simulink model "VTOL_renewal"  (R2023b)
settings: configuration reference "VTOLConfiguration" (kept outside this file)
undefined symbols (not defined in the file): CityMission, control, controlParams, ControlSampleTime, CriticalTiltAngle, DiscIntNeverNeededParam, env, F, FixedWingMission, flightState, FSState, FWControlParams, FWTrimSpeed, HoverMission, iniRoll, initPitch, iniYaw, Light, MIL, R_LOOKAHEAD, ReferenceFilterDen, ReferenceFilterNum, tilt_max, tilt_trim, tiltIni, TiltScheduleRate, TransitionMission, uavParam, vIni, Vt, w_trim, WindDownRate, windVel, xGround, yGround, zGround
libraries: slpidlib x56, simulink x6, uavalgslib x6, mbdriLib x4, aerolibasang x2, aerolibwind2 x2, shared6dof x1, sharedtransform x1, simulink_extras x1, sim3dlib x1, uavsim3dlib x1, uavutilslib x1
(part 1 of 8)
settings Model: DataDictionary=VTOLDynamicsData.sldd  Creator=The MathWorks, Inc.  LastModifiedBy=USER
settings ConfigSetRef: SourceName=VTOLConfiguration

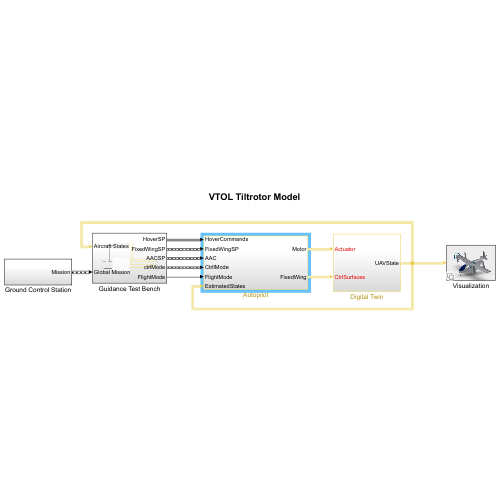
[thumbnail: Simulink's stored preview of the top-level diagram]
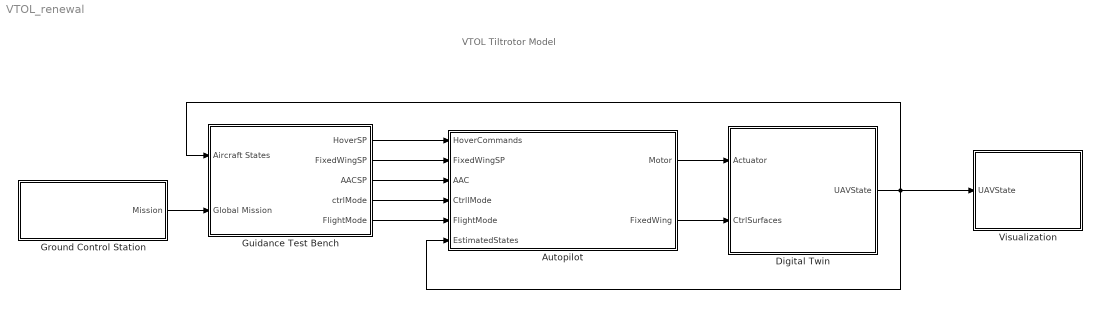
== system VTOL_renewal ==
  note: VTOL Tiltrotor Model
  Autopilot : Subsystem
  Digital Twin : Subsystem
  Ground Control Station : Subsystem
  Guidance Test Bench : Subsystem
  Visualization : Subsystem  Variant=on  VariantControl=Visualization
      mask Display: image('TiltrotorVisualization.PNG'); % Use "Edit Image" on toolstrip to change.
  wires:
  Autopilot/1(Motor) -> Digital Twin/1(Actuator)
  Autopilot/2(FixedWing) -> Digital Twin/2(CtrlSurfaces)
  Guidance Test Bench/1(HoverSP) -> Autopilot/1(HoverCommands)
  Ground Control Station/1(Mission) -> Guidance Test Bench/2(Global Mission)
  Guidance Test Bench/2(FixedWingSP) -> Autopilot/2(FixedWingSP)
  Guidance Test Bench/3(AACSP) -> Autopilot/3(AAC)
  Guidance Test Bench/5(FlightMode) -> Autopilot/5(FlightMode)
  Digital Twin/1(UAVState) -> Guidance Test Bench/1(Aircraft States), Autopilot/6(EstimatedStates), Visualization/1(UAVState)
  Guidance Test Bench/4(ctrlMode) -> Autopilot/4(CtrllMode)

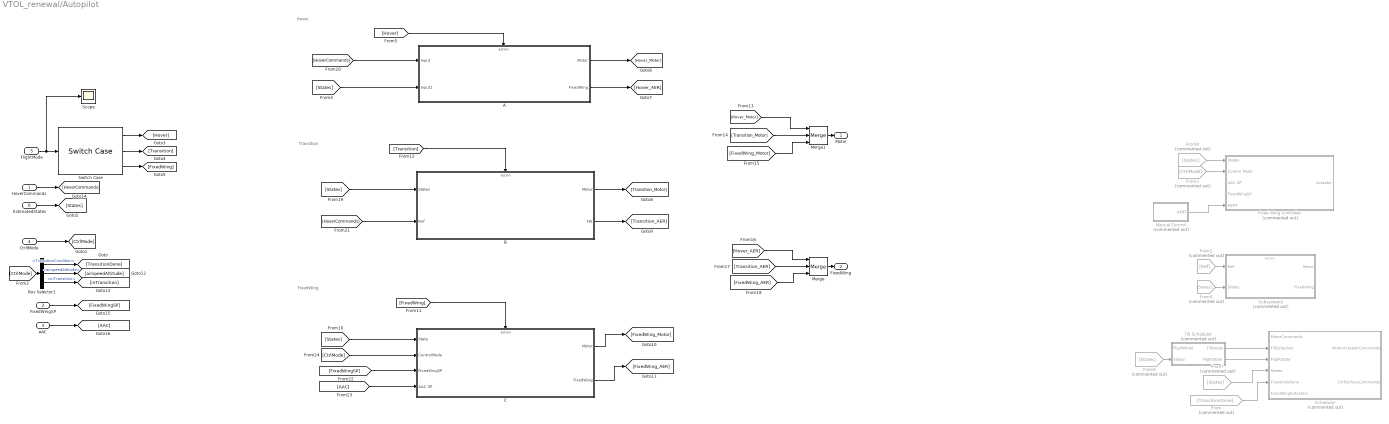
== system VTOL_renewal/Autopilot ==
  note: FixedWing
  note: Transition
  note: Hover
  HoverCommands : Inport
  FixedWingSP : Inport  Port=2
  AAC : Inport  Port=3
  CtrllMode : Inport  Port=4
  FlightMode : Inport  Port=5
  EstimatedStates : Inport  Port=6
  A : Subsystem  TreatAsAtomicUnit=on
  B : Subsystem
  Bus Selector1 : BusSelector  OutputSignals=TransitionCondition,airspeedAltitude,inTransition
  C : Subsystem
  Fixed Wing Controller : Subsystem  Commented=on  Variant=on  VariantControl=Fixed Wing Controller
  From : From  Commented=on  GotoTag=TransitionDone
  From1 : From  Commented=on  GotoTag=Ref
  From3 : From  Commented=on  GotoTag=CtrlMode
  From{6..9} (4 alike) : From  Commented=on  GotoTag=States
  Manual Control : Subsystem  Commented=on
  Merge : Merge  Inputs=3
  Merge1 : Merge  Inputs=3
  Scheduler : Subsystem  Commented=on  SystemSampleTime=0.005
  Scope : Scope
  Subsystem5 : Subsystem  Commented=on
  Switch Case : SwitchCase  CaseConditions={flightState.Hover, flightState.Transition, flightState.FixedWing}  ShowDefaultCase=off
  Tilt Scheduler : Subsystem  Commented=on
  Motor : Outport  OutDataTypeStr=Bus: RotorCntrlBus
  FixedWing : Outport  Port=2
  wires:
  Tilt Scheduler/1(TiltAngle) -> Scheduler/2(TiltSchedule)
  Manual Control/1(AERT) -> Fixed Wing Controller/5(AERT)
  From/1 -> Scheduler/5(TransitionDone)
  Tilt Scheduler/2(FlightState) -> Scheduler/3(FlightState)
  Bus Selector1/1 -> [TransitionDone]  "<TransitionCondition>"
  From3/1 -> Fixed Wing Controller/2(Control Mode)
  [CtrlMode] -> Bus Selector1/1
  EstimatedStates/1 -> [States]
  From8/1 -> Fixed Wing Controller/1(States)
  From6/1 -> Tilt Scheduler/2(States)
  From7/1 -> Scheduler/4(States)
  FlightMode/1 -> Scope/1, Switch Case/1
  Switch Case/1 -> [Hover]
  Switch Case/2 -> [Transition]
  Switch Case/3 -> [FixedWing]
  CtrllMode/1 -> [CtrlMode]
  From9/1 -> Subsystem5/2(States)
  From1/1 -> Subsystem5/1(Ref)
  [States] -> C/1(State)
  [Hover] -> A/Action
  [States] -> A/2(Input1)
  [Transition] -> B/Action
  A/1(Motor) -> [Hover_Motor]
  A/2(FixedWing) -> [Hover_AER]
  B/1(Motor) -> [Transition_Motor]
  B/2(FW) -> [Transition_AER]
  C/1(Motor) -> [FixedWing_Motor]
  C/2(FixedWing) -> [FixedWing_AER]
  [Transition_Motor] -> Merge1/2
  [Transition_AER] -> Merge/2
  [States] -> B/1(States)
  [FixedWing] -> C/Action
  Bus Selector1/2 -> [airspeedAltitude]  "<airspeedAltitude>"
  Bus Selector1/3 -> [inTransition]  "<inTransition>"
  FixedWingSP/1 -> [FixedWingSP]
  [Hover_Motor] -> Merge1/1
  [Hover_AER] -> Merge/1
  HoverCommands/1 -> [HoverCommands]
  [HoverCommands] -> A/1(Input)
  [HoverCommands] -> B/2(Ref)
  AAC/1 -> [AAC]
  [AAC] -> C/4(AAC SP)
  [FixedWingSP] -> C/3(FixedWingSP)
  [CtrlMode] -> C/2(ControlMode)
  Merge1/1 -> Motor/1
  [FixedWing_Motor] -> Merge1/3
  Merge/1 -> FixedWing/1
  [FixedWing_AER] -> Merge/3

== system VTOL_renewal/Digital Twin ==
  Actuator : Inport
  CtrlSurfaces : Inport  Port=2
  6DOF (Euler Angles)1 : shared6dof/6DOF (Euler Angles)  units=Metric (MKS)  mtype=Fixed  rep=Euler Angles  xme_0=[xGround, yGround, zGround]  Vm_0=[vIni 0 0]  eul_0=[iniRoll initPitch iniYaw]  pm_0=[0 0 0]  mass_0=6.031  mass_e=0.5  mass_f=2.0  inertia=[uavParam.geom.Ixx 0 0; 0 uavParam.geom.Iyy 0; 0 0 uavParam.geom.Izz]  inertia_e=eye(3)  inertia_f=2*eye(3)  k_quat=1.0  vre_flag=on  abi_flag=on  aMode=0  xme_statename=''  Vm_statename=''  eul_statename=''  quat_statename=''  pm_statename=''  mass_statename=''
  Bus Selector : BusSelector  OutputSignals=RotorParameters.w1,RotorParameters.w2,RotorParameters.w3,RotorParameters.w4
  Bus Selector1 : BusSelector  OutputSignals=Xe,Ve,Euler,pqr
  Demux : Demux  Outputs=3
  Demux1 : Demux  Outputs=3
  Force and Moments : Subsystem
  Ground Truth Bus : Subsystem
  Scope : Scope  NumInputPorts=4
  Scope{1..10} (10 alike) : Scope
  Subsystem2 : Subsystem
  Terminator : Terminator
  UAVState : Outport
  wires:
  Force and Moments/1(F) -> 6DOF (Euler Angles)1/1
  Force and Moments/2(M) -> 6DOF (Euler Angles)1/2
  Actuator/1 -> Force and Moments/1(Actuator)
  CtrlSurfaces/1 -> Force and Moments/2(CtrlSurfaces)
  6DOF (Euler Angles)1/1 -> Ground Truth Bus/1(Ve)  "Ve"
  6DOF (Euler Angles)1/2 -> Ground Truth Bus/2(Xe)  "Xe"
  6DOF (Euler Angles)1/3 -> Ground Truth Bus/3(Euler)  "Euler"
  6DOF (Euler Angles)1/4 -> Ground Truth Bus/4(DCMbe)  "DCMbe"
  6DOF (Euler Angles)1/5 -> Ground Truth Bus/5(Vb)  "Vb"
  6DOF (Euler Angles)1/6 -> Ground Truth Bus/6(pqr)  "pqr"
  6DOF (Euler Angles)1/7 -> Terminator/1
  6DOF (Euler Angles)1/8 -> Ground Truth Bus/7(Abb)  "Abb"
  Force and Moments/3(RotorParams) -> Ground Truth Bus/9(RotorParams)  "RotorParams"
  Force and Moments/4(AirData) -> Ground Truth Bus/10(AirData)
  6DOF (Euler Angles)1/9 -> Ground Truth Bus/8(Abe)
  Ground Truth Bus/1(Ground Truth) -> Bus Selector1/1, Bus Selector/1, UAVState/1, Force and Moments/3(States)  "Ground Truth"
  Bus Selector/1 -> Scope/1  "<w1>"
  Bus Selector/2 -> Scope/2  "<w2>"
  Bus Selector/3 -> Scope/3  "<w3>"
  Bus Selector/4 -> Scope/4  "<w4>"
  Bus Selector1/1 -> Scope1/1  "<Xe>"
  Bus Selector1/2 -> Scope2/1  "<Ve>"
  Bus Selector1/3 -> Subsystem2/1(Euler), Scope3/1, Demux/1  "<Euler>"
  Bus Selector1/4 -> Subsystem2/2(pqr), Scope4/1  "<pqr>"
  Demux/1 -> Scope5/1
  Demux/2 -> Scope6/1
  Demux/3 -> Scope7/1
  Subsystem2/1(Euler Rate) -> Demux1/1  "angRate"
  Demux1/1 -> Scope8/1
  Demux1/3 -> Scope10/1
  Demux1/2 -> Scope9/1

== system VTOL_renewal/Ground Control Station ==
  note: uavPathManagerBus type
  No Mission : Constant  Value=struct('mode',0,'position',[0 0 0]','params',[0;0;0;0]);  OutDataTypeStr=Bus: doubleUavPathManager
  Variant Source : VariantSource
  Waypoints : Constant  Value=FixedWingMission  OutDataTypeStr=Bus: doubleUavPathManager  SampleTime=-1
  Waypoints1 : Constant  Value=HoverMission  OutDataTypeStr=Bus: doubleUavPathManager  SampleTime=-1
  Waypoints2 : Constant  Value=TransitionMission  OutDataTypeStr=Bus: doubleUavPathManager  SampleTime=-1
  Waypoints3 : Constant  Value=CityMission  OutDataTypeStr=Bus: doubleUavPathManager  SampleTime=-1
  Mission : Outport
  wires:
  No Mission/1 -> Variant Source/1
  Waypoints2/1 -> Variant Source/4
  Variant Source/1 -> Mission/1
  Waypoints/1 -> Variant Source/2
  Waypoints1/1 -> Variant Source/3
  Waypoints3/1 -> Variant Source/5

== system VTOL_renewal/Guidance Test Bench ==
  Aircraft States : Inport
  Global Mission : Inport  Port=2
  ControlType : Subsystem  Variant=on  VariantControl=Choice
  Rate Transition : RateTransition  OutPortSampleTime=0.005
  "Reference Tracking " : Subsystem
      settings: PortSchema="{\"entries\":[{\"content\":{\"sides\":[{\"content\":{\"connectorIds\":[\"In1\"]},\"type\":\"ConnectorPlacement.EquallySpacedRectSide\",\"uuid\":\"259d5f1e-a362-4dc0-8429-ef92dd781b31\"},{\"content\":{\"connectorIds\":[\"In2\",\"In3\"],\"side\":\"RIGHT\"},\"type\":\"ConnectorPlacement.EquallySpacedRectSide\",\"uuid\":\"8f699bfb-ab92-4bfa-94de-3c6c350a8a94\"},{\"content\":{\"connectorIds\":[],\"side\":\"TOP\"},\"type\":\"ConnectorPlacement.EquallySpacedRectSide\",\"uuid\":\"95dbffc6-e5b7-446a-adcb-afa0cff8c552\"}]},\"type\":\"ConnectorPlacement.EquallySpacedConnector\",\"uuid\":\"e657b5d9-4fa5-41f8-85e3-18a1074ff1cd\"}],\"packageUris\":[\"http://schema.mathworks.com/mf0/Connector/R2020b\"],\"version\":\"1.0\"}"
  HoverSP : Outport
  FixedWingSP : Outport  Port=2
  AACSP : Outport  Port=3
  ctrlMode : Outport  Port=4
  FlightMode : Outport  Port=5
  wires:
  Aircraft States/1 -> Rate Transition/1
  Global Mission/1 -> ControlType/2(Global Mission)
  ControlType/2(FixedWingSP) -> FixedWingSP/1
  ControlType/5(FlightMode) -> FlightMode/1
  ControlType/4(ctrlMode) -> ctrlMode/1
  Rate Transition/1 -> "Reference Tracking "/1(State), ControlType/1(Aircraft States)
  ControlType/3(AACSP) -> "Reference Tracking "/3(AAC Commands), AACSP/1
  ControlType/1(HoverCmds) -> "Reference Tracking "/2(Position Command), HoverSP/1

== system VTOL_renewal/Visualization ==
  UAVState : Inport
  No Visualization : Subsystem  VariantControl=Visualization==0
  Photorealistic : Subsystem  VariantControl=Visualization==2
  Visualization : Subsystem  VariantControl=Visualization==1

== system VTOL_renewal/Autopilot/A ==
  Input : Inport
  Input1 : Inport  Port=2
  Action Port : ActionPort  ActionPortLabel=case [ Hover ]:
  Hover Control : Subsystem  TreatAsAtomicUnit=on
  Multicopter Controller : Subsystem
  Motor : Outport
  FixedWing : Outport  Port=2
  wires:
  Multicopter Controller/1(MixerCommands) -> Hover Control/1(MixerCommands)
  Hover Control/2(FW) -> FixedWing/1
  Input/1 -> Multicopter Controller/1(Hover Commands)
  Input1/1 -> Multicopter Controller/2(States)
  Hover Control/1(Motor) -> Motor/1

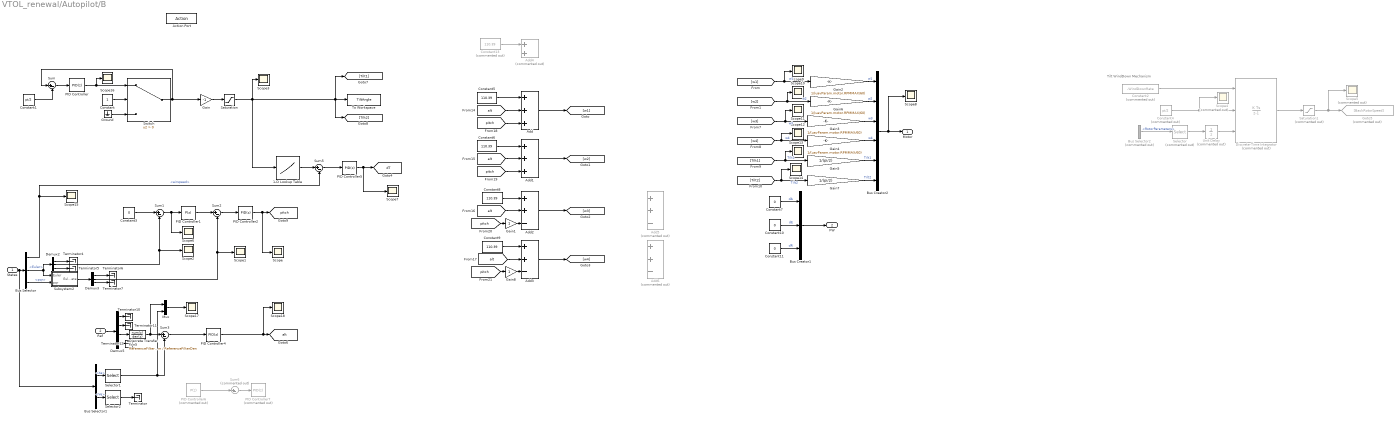
== system VTOL_renewal/Autopilot/B ==
  note: Tilt WindDown Mechanism
  States : Inport
  Ref : Inport  Port=2
  Action Port : ActionPort  ActionPortLabel=case [ Transition ]:
  1-D Lookup Table : Lookup_n-D  NumberOfTableDimensions=1  BreakpointsForDimension1=[-5:5]  Table=tanh([-5:5])  InternalRulePriority=Speed  RndMeth=Simplest
  Add : Sum  Inputs=+++
  Add1 : Sum  Inputs=+++
  Add2 : Sum  Inputs=++-
  Add3 : Sum  Inputs=++-
  Add4 : Sum  Commented=on
  Add5 : Sum  Commented=on  Inputs=++-
  Add6 : Sum  Commented=on  Inputs=++-
  Bus Creator1 : BusCreator  Inputs=3
  Bus Creator2 : BusCreator  Inputs=6  OutDataTypeStr=Bus: RotorCntrlBus
  Bus Selector : BusSelector  OutputSignals=airspeed,Euler,pqr
  Bus Selector1 : BusSelector  OutputSignals=Xe,Ve
  Bus Selector2 : BusSelector  Commented=on  OutputSignals=RotorParameters
  Constant : Constant
  Constant1 : Constant  Value=pi/2
  Constant{3,7,10..11} (4 alike) : Constant  Value=0
  Constant13 : Constant  Commented=on  Value=110.39
  Constant2 : Constant  Commented=on  Value=-WindDownRate
  Constant4 : Constant  Commented=on  Value=pi/2
  Constant{5..6,8..9} (4 alike) : Constant  Value=110.39
  Demux2 : Demux  Outputs=3
  Demux3 : Demux  Outputs=3
  Demux5 : Demux
  Discrete Transfer Fcn5 : DiscreteTransferFcn  Numerator=ReferenceFilterNum  Denominator=ReferenceFilterDen
  Discrete-Time Integrator : DiscreteIntegrator  Commented=on  ExternalReset=either  InitialConditionSource=external  SampleTime=0.005  ICPrevOutput=DiscIntNeverNeededParam  ICPrevScaledInput=DiscIntNeverNeededParam
  Gain : Gain  Gain=-1
  Gain1 : Gain
  Gain{2..4,6} (4 alike) : Gain  Gain=1/(uavParam.motor.RPMMAX/60)
  Gain5 : Gain  Gain=1/(pi/2)
  Gain7 : Gain  Gain=1/(pi/2)
  Gain8 : Gain
  Goto5 : Goto  Commented=on  GotoTag=BackRotorSpeed
  Ground : Ground
  Mux : Mux  Inputs=2
  PID Controller : slpidlib/PID Controller  Controller=PID  Form=Parallel  TimeDomain=Discrete-time  UseExternalTs=off  SampleTime=-1  IntegratorMethod=Forward Euler  FilterMethod=Forward Euler  ControllerParametersSource=internal  P=0  I=0.05  UseKiTs=off  D=0  N=100  UseFilter=on  TunerSelectOption=Transfer Function Based (PID Tuner App)  InitialConditionSource=internal  InitialConditionForIntegrator=0  InitialConditionForFilter=0  DifferentiatorICPrevScaledInput=0  ExternalReset=none  TrackingMode=off  Kt=1  LimitOutput=off  SatLimitsSource=internal  UpperSaturationLimit=inf  LowerSaturationLimit=-inf  LinearizeAsGain=on  AntiWindupMode=none  Kb=1  LimitIntegrator=off  UpperIntegratorSaturationLimit=inf  LowerIntegratorSaturationLimit=-inf  POutMin=[]  POutMax=[]  IOutMin=[]  IOutMax=[]  DOutMin=[]  DOutMax=[]  NOutMin=[]  NOutMax=[]  SumOutMin=[]  SumOutMax=[]  SaturationOutMin=[]  SaturationOutMax=[]  PParamMin=[]  PParamMax=[]  IParamMin=[]  IParamMax=[]  DParamMin=[]  DParamMax=[]  NParamMin=[]  NParamMax=[]  KbParamMin=[]  KbParamMax=[]  KtParamMin=[]  KtParamMax=[]  KbOutMin=[]  KbOutMax=[]  KtOutMin=[]  KtOutMax=[]  IntegratorOutMin=[]  IntegratorOutMax=[]  FilterOutMin=[]  FilterOutMax=[]  SumI1OutMin=[]  SumI1OutMax=[]  SumI2OutMin=[]  SumI2OutMax=[]  SumI3OutMin=[]  SumI3OutMax=[]  SumI4OutMin=[]  SumI4OutMax=[]  SumDOutMin=[]  SumDOutMax=[]  DifferentiatorOutMin=[]  DifferentiatorOutMax=[]  FilterDiffOutCoefMin=[]  FilterDiffOutCoefMax=[]  ReciprocalOutMin=[]  ReciprocalOutMax=[]  SumDenOutMin=[]  SumDenOutMax=[]  SumNumOutMin=[]  SumNumOutMax=[]  DivideOutMin=[]  DivideOutMax=[]  UdiffTsProdOutMin=[]  UdiffTsProdOutMax=[]  NTsProdOutMin=[]  NTsProdOutMax=[]  UintegralTsProdOutMin=[]  UintegralTsProdOutMax=[]  UngainTsProdOutMin=[]  UngainTsProdOutMax=[]  ClampingZeroOutDataTypeStr=Inherit: Inherit via back propagation  ClampingZeroOutMin=[]  ClampingZeroOutMax=[]  FilterDenConstantOutDataTypeStr=Inherit: Inherit via back propagation  FilterDenConstantOutMin=[]  FilterDenConstantOutMax=[]  PCopyOutDataTypeStr=Inherit: Inherit via back propagation  PCopyOutMin=[]  PCopyOutMax=[]  NCopyOutDataTypeStr=Inherit: Inherit via back propagation  NCopyOutMin=[]  NCopyOutMax=[]  IntegratorContinuousStateAttributes=''  IntegratorStateMustResolveToSignalObject=off  IntegratorRTWStateStorageClass=Auto  FilterContinuousStateAttributes=''  FilterStateMustResolveToSignalObject=off  FilterRTWStateStorageClass=Auto  ParallelPVariant=InternalParameters  IdealPVariant=Disabled  IVariant=InternalParameters  DVariant=InternalParameters  IntegratorVariant=Discrete  SatVariant=Disabled  AWVariant=Passthrough  PCopyVariant=Disabled  TRVariant=Disabled  FdbkBlocksVariant=Forward  IdealPFdbkVariant=Disabled  SatFdbkVariant=Disabled  DerivativeFilterVariant=ForwardEulerFilter  NVariant=InternalParameters  NCopyVariant=Disabled  FilterICVariant=InternalICsFilter  IntegratorICVariant=InternalICs  ExternalResetVariant=Disabled  TRSumVariant=Passthrough  SumFdbkVariant=Disabled  SumVariant=Sum_PID  TsampFilterVariant=InternalTs  TsampNgainVariant=Passthrough  TsampIntegralVariant=Disabled_SignalSpec  ExternalSaturationOutDataTypeStr=Inherit: Same as second input
  PID Controller1 : slpidlib/PID Controller  Controller=P  Form=Parallel  TimeDomain=Discrete-time  UseExternalTs=off  SampleTime=-1  IntegratorMethod=Forward Euler  FilterMethod=Forward Euler  ControllerParametersSource=internal  P=controlParams.P_PITCH  I=1  UseKiTs=off  D=0  N=100  UseFilter=on  TunerSelectOption=Transfer Function Based (PID Tuner App)  InitialConditionSource=internal  InitialConditionForIntegrator=0  InitialConditionForFilter=0  DifferentiatorICPrevScaledInput=0  ExternalReset=none  TrackingMode=off  Kt=1  LimitOutput=off  SatLimitsSource=internal  UpperSaturationLimit=inf  LowerSaturationLimit=-inf  LinearizeAsGain=on  AntiWindupMode=none  Kb=1  LimitIntegrator=off  UpperIntegratorSaturationLimit=inf  LowerIntegratorSaturationLimit=-inf  POutMin=[]  POutMax=[]  IOutMin=[]  IOutMax=[]  DOutMin=[]  DOutMax=[]  NOutMin=[]  NOutMax=[]  SumOutMin=[]  SumOutMax=[]  SaturationOutMin=[]  SaturationOutMax=[]  PParamMin=[]  PParamMax=[]  IParamMin=[]  IParamMax=[]  DParamMin=[]  DParamMax=[]  NParamMin=[]  NParamMax=[]  KbParamMin=[]  KbParamMax=[]  KtParamMin=[]  KtParamMax=[]  KbOutMin=[]  KbOutMax=[]  KtOutMin=[]  KtOutMax=[]  IntegratorOutMin=[]  IntegratorOutMax=[]  FilterOutMin=[]  FilterOutMax=[]  SumI1OutMin=[]  SumI1OutMax=[]  SumI2OutMin=[]  SumI2OutMax=[]  SumI3OutMin=[]  SumI3OutMax=[]  SumI4OutMin=[]  SumI4OutMax=[]  SumDOutMin=[]  SumDOutMax=[]  DifferentiatorOutMin=[]  DifferentiatorOutMax=[]  FilterDiffOutCoefMin=[]  FilterDiffOutCoefMax=[]  ReciprocalOutMin=[]  ReciprocalOutMax=[]  SumDenOutMin=[]  SumDenOutMax=[]  SumNumOutMin=[]  SumNumOutMax=[]  DivideOutMin=[]  DivideOutMax=[]  UdiffTsProdOutMin=[]  UdiffTsProdOutMax=[]  NTsProdOutMin=[]  NTsProdOutMax=[]  UintegralTsProdOutMin=[]  UintegralTsProdOutMax=[]  UngainTsProdOutMin=[]  UngainTsProdOutMax=[]  ClampingZeroOutDataTypeStr=Inherit: Inherit via back propagation  ClampingZeroOutMin=[]  ClampingZeroOutMax=[]  FilterDenConstantOutDataTypeStr=Inherit: Inherit via back propagation  FilterDenConstantOutMin=[]  FilterDenConstantOutMax=[]  PCopyOutDataTypeStr=Inherit: Inherit via back propagation  PCopyOutMin=[]  PCopyOutMax=[]  NCopyOutDataTypeStr=Inherit: Inherit via back propagation  NCopyOutMin=[]  NCopyOutMax=[]  IntegratorContinuousStateAttributes=''  IntegratorStateMustResolveToSignalObject=off  IntegratorRTWStateStorageClass=Auto  FilterContinuousStateAttributes=''  FilterStateMustResolveToSignalObject=off  FilterRTWStateStorageClass=Auto  ParallelPVariant=InternalParameters  IdealPVariant=Disabled  IVariant=Disabled  DVariant=Disabled  IntegratorVariant=Disabled  SatVariant=Disabled  AWVariant=Disabled  PCopyVariant=Disabled  TRVariant=Disabled  FdbkBlocksVariant=Forward  IdealPFdbkVariant=Disabled  SatFdbkVariant=Disabled  DerivativeFilterVariant=Disabled  NVariant=Disabled  NCopyVariant=Disabled_SignalSpec  FilterICVariant=Disabled  IntegratorICVariant=Disabled  ExternalResetVariant=Disabled  TRSumVariant=Passthrough  SumFdbkVariant=Disabled  SumVariant=Passthrough_P  TsampFilterVariant=InternalTs  TsampNgainVariant=Passthrough  TsampIntegralVariant=Disabled_SignalSpec  ExternalSaturationOutDataTypeStr=Inherit: Same as second input
  PID Controller2 : slpidlib/PID Controller  Controller=PID  Form=Parallel  TimeDomain=Discrete-time  UseExternalTs=off  SampleTime=-1  IntegratorMethod=Forward Euler  FilterMethod=Forward Euler  ControllerParametersSource=internal  P=controlParams.P_PITCH_RATE  I=controlParams.I_PITCH_RATE  UseKiTs=off  D=controlParams.D_PITCH_RATE  N=controlParams.N_PITCH_RATE  UseFilter=on  TunerSelectOption=Transfer Function Based (PID Tuner App)  InitialConditionSource=internal  InitialConditionForIntegrator=0  InitialConditionForFilter=0  DifferentiatorICPrevScaledInput=0  ExternalReset=none  TrackingMode=off  Kt=1  LimitOutput=off  SatLimitsSource=internal  UpperSaturationLimit=inf  LowerSaturationLimit=-inf  LinearizeAsGain=on  AntiWindupMode=none  Kb=1  LimitIntegrator=off  UpperIntegratorSaturationLimit=inf  LowerIntegratorSaturationLimit=-inf  POutMin=[]  POutMax=[]  IOutMin=[]  IOutMax=[]  DOutMin=[]  DOutMax=[]  NOutMin=[]  NOutMax=[]  SumOutMin=[]  SumOutMax=[]  SaturationOutMin=[]  SaturationOutMax=[]  PParamMin=[]  PParamMax=[]  IParamMin=[]  IParamMax=[]  DParamMin=[]  DParamMax=[]  NParamMin=[]  NParamMax=[]  KbParamMin=[]  KbParamMax=[]  KtParamMin=[]  KtParamMax=[]  KbOutMin=[]  KbOutMax=[]  KtOutMin=[]  KtOutMax=[]  IntegratorOutMin=[]  IntegratorOutMax=[]  FilterOutMin=[]  FilterOutMax=[]  SumI1OutMin=[]  SumI1OutMax=[]  SumI2OutMin=[]  SumI2OutMax=[]  SumI3OutMin=[]  SumI3OutMax=[]  SumI4OutMin=[]  SumI4OutMax=[]  SumDOutMin=[]  SumDOutMax=[]  DifferentiatorOutMin=[]  DifferentiatorOutMax=[]  FilterDiffOutCoefMin=[]  FilterDiffOutCoefMax=[]  ReciprocalOutMin=[]  ReciprocalOutMax=[]  SumDenOutMin=[]  SumDenOutMax=[]  SumNumOutMin=[]  SumNumOutMax=[]  DivideOutMin=[]  DivideOutMax=[]  UdiffTsProdOutMin=[]  UdiffTsProdOutMax=[]  NTsProdOutMin=[]  NTsProdOutMax=[]  UintegralTsProdOutMin=[]  UintegralTsProdOutMax=[]  UngainTsProdOutMin=[]  UngainTsProdOutMax=[]  ClampingZeroOutDataTypeStr=Inherit: Inherit via back propagation  ClampingZeroOutMin=[]  ClampingZeroOutMax=[]  FilterDenConstantOutDataTypeStr=Inherit: Inherit via back propagation  FilterDenConstantOutMin=[]  FilterDenConstantOutMax=[]  PCopyOutDataTypeStr=Inherit: Inherit via back propagation  PCopyOutMin=[]  PCopyOutMax=[]  NCopyOutDataTypeStr=Inherit: Inherit via back propagation  NCopyOutMin=[]  NCopyOutMax=[]  IntegratorContinuousStateAttributes=''  IntegratorStateMustResolveToSignalObject=off  IntegratorRTWStateStorageClass=Auto  FilterContinuousStateAttributes=''  FilterStateMustResolveToSignalObject=off  FilterRTWStateStorageClass=Auto  ParallelPVariant=InternalParameters  IdealPVariant=Disabled  IVariant=InternalParameters  DVariant=InternalParameters  IntegratorVariant=Discrete  SatVariant=Disabled  AWVariant=Passthrough  PCopyVariant=Disabled  TRVariant=Disabled  FdbkBlocksVariant=Forward  IdealPFdbkVariant=Disabled  SatFdbkVariant=Disabled  DerivativeFilterVariant=ForwardEulerFilter  NVariant=InternalParameters  NCopyVariant=Disabled  FilterICVariant=InternalICsFilter  IntegratorICVariant=InternalICs  ExternalResetVariant=Disabled  TRSumVariant=Passthrough  SumFdbkVariant=Disabled  SumVariant=Sum_PID  TsampFilterVariant=InternalTs  TsampNgainVariant=Passthrough  TsampIntegralVariant=Disabled_SignalSpec  ExternalSaturationOutDataTypeStr=Inherit: Same as second input
  PID Controller4 : slpidlib/PID Controller  Controller=PID  Form=Parallel  TimeDomain=Discrete-time  UseExternalTs=off  SampleTime=-1  IntegratorMethod=Forward Euler  FilterMethod=Forward Euler  ControllerParametersSource=internal  P=controlParams.P_VZ  I=controlParams.I_Z  UseKiTs=off  D=controlParams.D_VZ  N=controlParams.N_VZ  UseFilter=on  TunerSelectOption=Transfer Function Based (PID Tuner App)  InitialConditionSource=internal  InitialConditionForIntegrator=0  InitialConditionForFilter=0  DifferentiatorICPrevScaledInput=0  ExternalReset=none  TrackingMode=off  Kt=1  LimitOutput=off  SatLimitsSource=internal  UpperSaturationLimit=inf  LowerSaturationLimit=-inf  LinearizeAsGain=on  AntiWindupMode=none  Kb=1  LimitIntegrator=off  UpperIntegratorSaturationLimit=inf  LowerIntegratorSaturationLimit=-inf  POutMin=[]  POutMax=[]  IOutMin=[]  IOutMax=[]  DOutMin=[]  DOutMax=[]  NOutMin=[]  NOutMax=[]  SumOutMin=[]  SumOutMax=[]  SaturationOutMin=[]  SaturationOutMax=[]  PParamMin=[]  PParamMax=[]  IParamMin=[]  IParamMax=[]  DParamMin=[]  DParamMax=[]  NParamMin=[]  NParamMax=[]  KbParamMin=[]  KbParamMax=[]  KtParamMin=[]  KtParamMax=[]  KbOutMin=[]  KbOutMax=[]  KtOutMin=[]  KtOutMax=[]  IntegratorOutMin=[]  IntegratorOutMax=[]  FilterOutMin=[]  FilterOutMax=[]  SumI1OutMin=[]  SumI1OutMax=[]  SumI2OutMin=[]  SumI2OutMax=[]  SumI3OutMin=[]  SumI3OutMax=[]  SumI4OutMin=[]  SumI4OutMax=[]  SumDOutMin=[]  SumDOutMax=[]  DifferentiatorOutMin=[]  DifferentiatorOutMax=[]  FilterDiffOutCoefMin=[]  FilterDiffOutCoefMax=[]  ReciprocalOutMin=[]  ReciprocalOutMax=[]  SumDenOutMin=[]  SumDenOutMax=[]  SumNumOutMin=[]  SumNumOutMax=[]  DivideOutMin=[]  DivideOutMax=[]  UdiffTsProdOutMin=[]  UdiffTsProdOutMax=[]  NTsProdOutMin=[]  NTsProdOutMax=[]  UintegralTsProdOutMin=[]  UintegralTsProdOutMax=[]  UngainTsProdOutMin=[]  UngainTsProdOutMax=[]  ClampingZeroOutDataTypeStr=Inherit: Inherit via back propagation  ClampingZeroOutMin=[]  ClampingZeroOutMax=[]  FilterDenConstantOutDataTypeStr=Inherit: Inherit via back propagation  FilterDenConstantOutMin=[]  FilterDenConstantOutMax=[]  PCopyOutDataTypeStr=Inherit: Inherit via back propagation  PCopyOutMin=[]  PCopyOutMax=[]  NCopyOutDataTypeStr=Inherit: Inherit via back propagation  NCopyOutMin=[]  NCopyOutMax=[]  IntegratorContinuousStateAttributes=''  IntegratorStateMustResolveToSignalObject=off  IntegratorRTWStateStorageClass=Auto  FilterContinuousStateAttributes=''  FilterStateMustResolveToSignalObject=off  FilterRTWStateStorageClass=Auto  ParallelPVariant=InternalParameters  IdealPVariant=Disabled  IVariant=InternalParameters  DVariant=InternalParameters  IntegratorVariant=Discrete  SatVariant=Disabled  AWVariant=Passthrough  PCopyVariant=Disabled  TRVariant=Disabled  FdbkBlocksVariant=Forward  IdealPFdbkVariant=Disabled  SatFdbkVariant=Disabled  DerivativeFilterVariant=ForwardEulerFilter  NVariant=InternalParameters  NCopyVariant=Disabled  FilterICVariant=InternalICsFilter  IntegratorICVariant=InternalICs  ExternalResetVariant=Disabled  TRSumVariant=Passthrough  SumFdbkVariant=Disabled  SumVariant=Sum_PID  TsampFilterVariant=InternalTs  TsampNgainVariant=Passthrough  TsampIntegralVariant=Disabled_SignalSpec  ExternalSaturationOutDataTypeStr=Inherit: Same as second input
  PID Controller5 : slpidlib/PID Controller  Controller=PID  Form=Parallel  TimeDomain=Discrete-time  UseExternalTs=off  SampleTime=-1  IntegratorMethod=Forward Euler  FilterMethod=Forward Euler  ControllerParametersSource=internal  P=10  I=15  UseKiTs=off  D=0  N=100  UseFilter=on  TunerSelectOption=Transfer Function Based (PID Tuner App)  InitialConditionSource=internal  InitialConditionForIntegrator=0  InitialConditionForFilter=0  DifferentiatorICPrevScaledInput=0  ExternalReset=none  TrackingMode=off  Kt=1  LimitOutput=off  SatLimitsSource=internal  UpperSaturationLimit=inf  LowerSaturationLimit=-inf  LinearizeAsGain=on  AntiWindupMode=none  Kb=1  LimitIntegrator=off  UpperIntegratorSaturationLimit=inf  LowerIntegratorSaturationLimit=-inf  POutMin=[]  POutMax=[]  IOutMin=[]  IOutMax=[]  DOutMin=[]  DOutMax=[]  NOutMin=[]  NOutMax=[]  SumOutMin=[]  SumOutMax=[]  SaturationOutMin=[]  SaturationOutMax=[]  PParamMin=[]  PParamMax=[]  IParamMin=[]  IParamMax=[]  DParamMin=[]  DParamMax=[]  NParamMin=[]  NParamMax=[]  KbParamMin=[]  KbParamMax=[]  KtParamMin=[]  KtParamMax=[]  KbOutMin=[]  KbOutMax=[]  KtOutMin=[]  KtOutMax=[]  IntegratorOutMin=[]  IntegratorOutMax=[]  FilterOutMin=[]  FilterOutMax=[]  SumI1OutMin=[]  SumI1OutMax=[]  SumI2OutMin=[]  SumI2OutMax=[]  SumI3OutMin=[]  SumI3OutMax=[]  SumI4OutMin=[]  SumI4OutMax=[]  SumDOutMin=[]  SumDOutMax=[]  DifferentiatorOutMin=[]  DifferentiatorOutMax=[]  FilterDiffOutCoefMin=[]  FilterDiffOutCoefMax=[]  ReciprocalOutMin=[]  ReciprocalOutMax=[]  SumDenOutMin=[]  SumDenOutMax=[]  SumNumOutMin=[]  SumNumOutMax=[]  DivideOutMin=[]  DivideOutMax=[]  UdiffTsProdOutMin=[]  UdiffTsProdOutMax=[]  NTsProdOutMin=[]  NTsProdOutMax=[]  UintegralTsProdOutMin=[]  UintegralTsProdOutMax=[]  UngainTsProdOutMin=[]  UngainTsProdOutMax=[]  ClampingZeroOutDataTypeStr=Inherit: Inherit via back propagation  ClampingZeroOutMin=[]  ClampingZeroOutMax=[]  FilterDenConstantOutDataTypeStr=Inherit: Inherit via back propagation  FilterDenConstantOutMin=[]  FilterDenConstantOutMax=[]  PCopyOutDataTypeStr=Inherit: Inherit via back propagation  PCopyOutMin=[]  PCopyOutMax=[]  NCopyOutDataTypeStr=Inherit: Inherit via back propagation  NCopyOutMin=[]  NCopyOutMax=[]  IntegratorContinuousStateAttributes=''  IntegratorStateMustResolveToSignalObject=off  IntegratorRTWStateStorageClass=Auto  FilterContinuousStateAttributes=''  FilterStateMustResolveToSignalObject=off  FilterRTWStateStorageClass=Auto  ParallelPVariant=InternalParameters  IdealPVariant=Disabled  IVariant=InternalParameters  DVariant=InternalParameters  IntegratorVariant=Discrete  SatVariant=Disabled  AWVariant=Passthrough  PCopyVariant=Disabled  TRVariant=Disabled  FdbkBlocksVariant=Forward  IdealPFdbkVariant=Disabled  SatFdbkVariant=Disabled  DerivativeFilterVariant=ForwardEulerFilter  NVariant=InternalParameters  NCopyVariant=Disabled  FilterICVariant=InternalICsFilter  IntegratorICVariant=InternalICs  ExternalResetVariant=Disabled  TRSumVariant=Passthrough  SumFdbkVariant=Disabled  SumVariant=Sum_PID  TsampFilterVariant=InternalTs  TsampNgainVariant=Passthrough  TsampIntegralVariant=Disabled_SignalSpec  ExternalSaturationOutDataTypeStr=Inherit: Same as second input
  PID Controller6 : slpidlib/PID Controller  Commented=on  Controller=P  Form=Parallel  TimeDomain=Discrete-time  UseExternalTs=off  SampleTime=-1  IntegratorMethod=Forward Euler  FilterMethod=Forward Euler  ControllerParametersSource=internal  P=controlParams.P_Z  I=controlParams.I_Z  UseKiTs=off  D=controlParams.D_Z  N=controlParams.N_Z  UseFilter=on  TunerSelectOption=Transfer Function Based (PID Tuner App)  InitialConditionSource=internal  InitialConditionForIntegrator=0  InitialConditionForFilter=0  DifferentiatorICPrevScaledInput=0  ExternalReset=none  TrackingMode=off  Kt=1  LimitOutput=off  SatLimitsSource=internal  UpperSaturationLimit=inf  LowerSaturationLimit=-inf  LinearizeAsGain=on  AntiWindupMode=none  Kb=1  LimitIntegrator=off  UpperIntegratorSaturationLimit=inf  LowerIntegratorSaturationLimit=-inf  POutMin=[]  POutMax=[]  IOutMin=[]  IOutMax=[]  DOutMin=[]  DOutMax=[]  NOutMin=[]  NOutMax=[]  SumOutMin=[]  SumOutMax=[]  SaturationOutMin=[]  SaturationOutMax=[]  PParamMin=[]  PParamMax=[]  IParamMin=[]  IParamMax=[]  DParamMin=[]  DParamMax=[]  NParamMin=[]  NParamMax=[]  KbParamMin=[]  KbParamMax=[]  KtParamMin=[]  KtParamMax=[]  KbOutMin=[]  KbOutMax=[]  KtOutMin=[]  KtOutMax=[]  IntegratorOutMin=[]  IntegratorOutMax=[]  FilterOutMin=[]  FilterOutMax=[]  SumI1OutMin=[]  SumI1OutMax=[]  SumI2OutMin=[]  SumI2OutMax=[]  SumI3OutMin=[]  SumI3OutMax=[]  SumI4OutMin=[]  SumI4OutMax=[]  SumDOutMin=[]  SumDOutMax=[]  DifferentiatorOutMin=[]  DifferentiatorOutMax=[]  FilterDiffOutCoefMin=[]  FilterDiffOutCoefMax=[]  ReciprocalOutMin=[]  ReciprocalOutMax=[]  SumDenOutMin=[]  SumDenOutMax=[]  SumNumOutMin=[]  SumNumOutMax=[]  DivideOutMin=[]  DivideOutMax=[]  UdiffTsProdOutMin=[]  UdiffTsProdOutMax=[]  NTsProdOutMin=[]  NTsProdOutMax=[]  UintegralTsProdOutMin=[]  UintegralTsProdOutMax=[]  UngainTsProdOutMin=[]  UngainTsProdOutMax=[]  ClampingZeroOutDataTypeStr=Inherit: Inherit via back propagation  ClampingZeroOutMin=[]  ClampingZeroOutMax=[]  FilterDenConstantOutDataTypeStr=Inherit: Inherit via back propagation  FilterDenConstantOutMin=[]  FilterDenConstantOutMax=[]  PCopyOutDataTypeStr=Inherit: Inherit via back propagation  PCopyOutMin=[]  PCopyOutMax=[]  NCopyOutDataTypeStr=Inherit: Inherit via back propagation  NCopyOutMin=[]  NCopyOutMax=[]  IntegratorContinuousStateAttributes=''  IntegratorStateMustResolveToSignalObject=off  IntegratorRTWStateStorageClass=Auto  FilterContinuousStateAttributes=''  FilterStateMustResolveToSignalObject=off  FilterRTWStateStorageClass=Auto  ParallelPVariant=InternalParameters  IdealPVariant=Disabled  IVariant=Disabled  DVariant=Disabled  IntegratorVariant=Disabled  SatVariant=Disabled  AWVariant=Disabled  PCopyVariant=Disabled  TRVariant=Disabled  FdbkBlocksVariant=Forward  IdealPFdbkVariant=Disabled  SatFdbkVariant=Disabled  DerivativeFilterVariant=Disabled  NVariant=Disabled  NCopyVariant=Disabled_SignalSpec  FilterICVariant=Disabled  IntegratorICVariant=Disabled  ExternalResetVariant=Disabled  TRSumVariant=Passthrough  SumFdbkVariant=Disabled  SumVariant=Passthrough_P  TsampFilterVariant=InternalTs  TsampNgainVariant=Passthrough  TsampIntegralVariant=Disabled_SignalSpec  ExternalSaturationOutDataTypeStr=Inherit: Same as second input
  PID Controller7 : slpidlib/PID Controller  Commented=on  Controller=PID  Form=Parallel  TimeDomain=Discrete-time  UseExternalTs=off  SampleTime=-1  IntegratorMethod=Forward Euler  FilterMethod=Forward Euler  ControllerParametersSource=internal  P=controlParams.P_VZ  I=controlParams.I_Z  UseKiTs=off  D=controlParams.D_VZ  N=controlParams.N_VZ  UseFilter=on  TunerSelectOption=Transfer Function Based (PID Tuner App)  InitialConditionSource=internal  InitialConditionForIntegrator=0  InitialConditionForFilter=0  DifferentiatorICPrevScaledInput=0  ExternalReset=none  TrackingMode=off  Kt=1  LimitOutput=off  SatLimitsSource=internal  UpperSaturationLimit=inf  LowerSaturationLimit=-inf  LinearizeAsGain=on  AntiWindupMode=none  Kb=1  LimitIntegrator=off  UpperIntegratorSaturationLimit=inf  LowerIntegratorSaturationLimit=-inf  POutMin=[]  POutMax=[]  IOutMin=[]  IOutMax=[]  DOutMin=[]  DOutMax=[]  NOutMin=[]  NOutMax=[]  SumOutMin=[]  SumOutMax=[]  SaturationOutMin=[]  SaturationOutMax=[]  PParamMin=[]  PParamMax=[]  IParamMin=[]  IParamMax=[]  DParamMin=[]  DParamMax=[]  NParamMin=[]  NParamMax=[]  KbParamMin=[]  KbParamMax=[]  KtParamMin=[]  KtParamMax=[]  KbOutMin=[]  KbOutMax=[]  KtOutMin=[]  KtOutMax=[]  IntegratorOutMin=[]  IntegratorOutMax=[]  FilterOutMin=[]  FilterOutMax=[]  SumI1OutMin=[]  SumI1OutMax=[]  SumI2OutMin=[]  SumI2OutMax=[]  SumI3OutMin=[]  SumI3OutMax=[]  SumI4OutMin=[]  SumI4OutMax=[]  SumDOutMin=[]  SumDOutMax=[]  DifferentiatorOutMin=[]  DifferentiatorOutMax=[]  FilterDiffOutCoefMin=[]  FilterDiffOutCoefMax=[]  ReciprocalOutMin=[]  ReciprocalOutMax=[]  SumDenOutMin=[]  SumDenOutMax=[]  SumNumOutMin=[]  SumNumOutMax=[]  DivideOutMin=[]  DivideOutMax=[]  UdiffTsProdOutMin=[]  UdiffTsProdOutMax=[]  NTsProdOutMin=[]  NTsProdOutMax=[]  UintegralTsProdOutMin=[]  UintegralTsProdOutMax=[]  UngainTsProdOutMin=[]  UngainTsProdOutMax=[]  ClampingZeroOutDataTypeStr=Inherit: Inherit via back propagation  ClampingZeroOutMin=[]  ClampingZeroOutMax=[]  FilterDenConstantOutDataTypeStr=Inherit: Inherit via back propagation  FilterDenConstantOutMin=[]  FilterDenConstantOutMax=[]  PCopyOutDataTypeStr=Inherit: Inherit via back propagation  PCopyOutMin=[]  PCopyOutMax=[]  NCopyOutDataTypeStr=Inherit: Inherit via back propagation  NCopyOutMin=[]  NCopyOutMax=[]  IntegratorContinuousStateAttributes=''  IntegratorStateMustResolveToSignalObject=off  IntegratorRTWStateStorageClass=Auto  FilterContinuousStateAttributes=''  FilterStateMustResolveToSignalObject=off  FilterRTWStateStorageClass=Auto  ParallelPVariant=InternalParameters  IdealPVariant=Disabled  IVariant=InternalParameters  DVariant=InternalParameters  IntegratorVariant=Discrete  SatVariant=Disabled  AWVariant=Passthrough  PCopyVariant=Disabled  TRVariant=Disabled  FdbkBlocksVariant=Forward  IdealPFdbkVariant=Disabled  SatFdbkVariant=Disabled  DerivativeFilterVariant=ForwardEulerFilter  NVariant=InternalParameters  NCopyVariant=Disabled  FilterICVariant=InternalICsFilter  IntegratorICVariant=InternalICs  ExternalResetVariant=Disabled  TRSumVariant=Passthrough  SumFdbkVariant=Disabled  SumVariant=Sum_PID  TsampFilterVariant=InternalTs  TsampNgainVariant=Passthrough  TsampIntegralVariant=Disabled_SignalSpec  ExternalSaturationOutDataTypeStr=Inherit: Same as second input
  Saturation : Saturate  UpperLimit=pi/2  LowerLimit=0
  Saturation1 : Saturate  Commented=on  UpperLimit=Inf  LowerLimit=0
  Scope{,1..3,6..18} (17 alike) : Scope
  Scope4 : Scope  Commented=on
  Scope5 : Scope  Commented=on
  Selector : Selector  Commented=on  InputPortWidth=6  IndexOptions=Index vector (dialog)  Indices=4  OutputSizes=1
  Selector1 : Selector  InputPortWidth=3  IndexOptions=Index vector (dialog)  Indices=[3]  OutputSizes=1
  Selector2 : Selector  InputPortWidth=3  IndexOptions=Index vector (dialog)  Indices=[3]  OutputSizes=1
  Subsystem2 : Subsystem
  Sum{,1..3,5} (5 alike) : Sum  Inputs=|+-
  Sum6 : Sum  Commented=on  Inputs=|+-
  Switch : Switch  Criteria=u2 > Threshold  SaturateOnIntegerOverflow=off  InputSameDT=off
  Terminator{,4..7,10..12} (8 alike) : Terminator
  To Workspace : ToWorkspace  VariableName=TiltAngle  SampleTime=-1
  Unit Delay : UnitDelay  Commented=on  SampleTime=-1  HasFrameUpgradeWarning=on
  Motor : Outport
  FW : Outport  Port=2
  tag scope: alt=global, dT=global, pitch=global
  wires:
  [w1] -> Scope9/1, Gain2/1  "w1"
  [w2] -> Scope10/1, Gain6/1  "w2"
  [w3] -> Scope11/1, Gain3/1  "w3"
  [w4] -> Gain4/1, Scope12/1  "w4"
  [Tilt1] -> Scope13/1, Gain5/1  "Tilt1"
  [Tilt2] -> Gain7/1, Scope14/1  "Tilt2"
  Constant10/1 -> Bus Creator1/2  "dE"
  Constant11/1 -> Bus Creator1/3  "dR"
  Constant7/1 -> Bus Creator1/1  "dA"
  Bus Creator1/1 -> FW/1
  Bus Selector/2 -> Subsystem2/1(Euler), Demux2/1  "<Euler>"
  Demux2/3 -> Terminator5/1
  Demux2/1 -> Terminator4/1
  Demux3/1 -> Terminator6/1
  Demux3/3 -> Terminator7/1
  Constant3/1 -> Sum1/1
  Demux2/2 -> Scope2/1, Sum1/2
  Sum1/1 -> Scope6/1, PID Controller1/1
  PID Controller1/1 -> Sum2/1
  Demux3/2 -> Sum2/2, Scope1/1
  Sum2/1 -> PID Controller2/1
  PID Controller2/1 -> [pitch], Scope/1
  Constant/1 -> Switch/2
  Ground/1 -> Switch/3
  Switch/1 -> Sum/1, Gain/1
  Constant1/1 -> Sum/2
  Sum/1 -> PID Controller/1
  Gain/1 -> Saturation/1
  PID Controller/1 -> Scope16/1, Switch/1
  Saturation/1 -> 1-D Lookup Table/1, To Workspace/1, [Tilt2], [Tilt1], Scope3/1
  Constant2/1 -> Discrete-Time Integrator/1
  Unit Delay/1 -> Discrete-Time Integrator/3
  Saturation1/1 -> Scope5/1, Goto5/1
  Discrete-Time Integrator/1 -> Saturation1/1
  Bus Selector2/1 -> Selector/1  "<RotorParameters>"
  Selector/1 -> Unit Delay/1
  Constant4/1 -> Scope4/1, Discrete-Time Integrator/2
  Gain4/1 -> Bus Creator2/4  "w4"
  Bus Creator2/1 -> Scope8/1, Motor/1
  Gain7/1 -> Bus Creator2/6  "Tilt2"
  Gain5/1 -> Bus Creator2/5  "Tilt1"
  Gain3/1 -> Bus Creator2/3  "w3"
  Gain2/1 -> Bus Creator2/1  "w1"
  Gain6/1 -> Bus Creator2/2  "w2"
  Subsystem2/1(Euler Rate) -> Demux3/1
  Bus Selector/3 -> Subsystem2/2(pqr)  "<pqr>"
  [alt] -> Add2/2
  Add/1 -> [w1]
  Constant6/1 -> Add1/1
  Add2/1 -> [w3]
  Add3/1 -> [w4]
  [alt] -> Add/2
  Constant8/1 -> Add2/1
  Add1/1 -> [w2]
  Constant5/1 -> Add/1
  Constant9/1 -> Add3/1
  [pitch] -> Add/3
  [alt] -> Add3/2
  [alt] -> Add1/2
  Bus Selector1/1 -> Selector1/1  "<Xe>"
  Selector1/1 -> Mux/2, Sum3/2
  Bus Selector1/2 -> Selector2/1  "<Ve>"
  Sum3/1 -> PID Controller4/1
  PID Controller4/1 -> Scope18/1, [alt]
  States/1 -> Bus Selector1/1, Bus Selector/1
  [pitch] -> Add1/3
  Ref/1 -> Demux5/1
  Demux5/1 -> Terminator10/1
  Demux5/2 -> Terminator11/1
  Demux5/4 -> Terminator12/1
  Demux5/3 -> Discrete Transfer Fcn5/1
  Discrete Transfer Fcn5/1 -> Mux/1, Sum3/1
  1-D Lookup Table/1 -> Sum5/1
  Bus Selector/1 -> Sum5/2, Scope15/1  "<airspeed>"
  Sum5/1 -> PID Controller5/1
  PID Controller5/1 -> Scope7/1, [dT]
  Constant13/1 -> Add4/1
  [pitch] -> Gain8/1
  Gain8/1 -> Add3/3
  Gain1/1 -> Add2/3
  [pitch] -> Gain1/1
  Mux/1 -> Scope17/1
  Selector2/1 -> Terminator/1
  Sum6/1 -> PID Controller7/1
  PID Controller6/1 -> Sum6/1

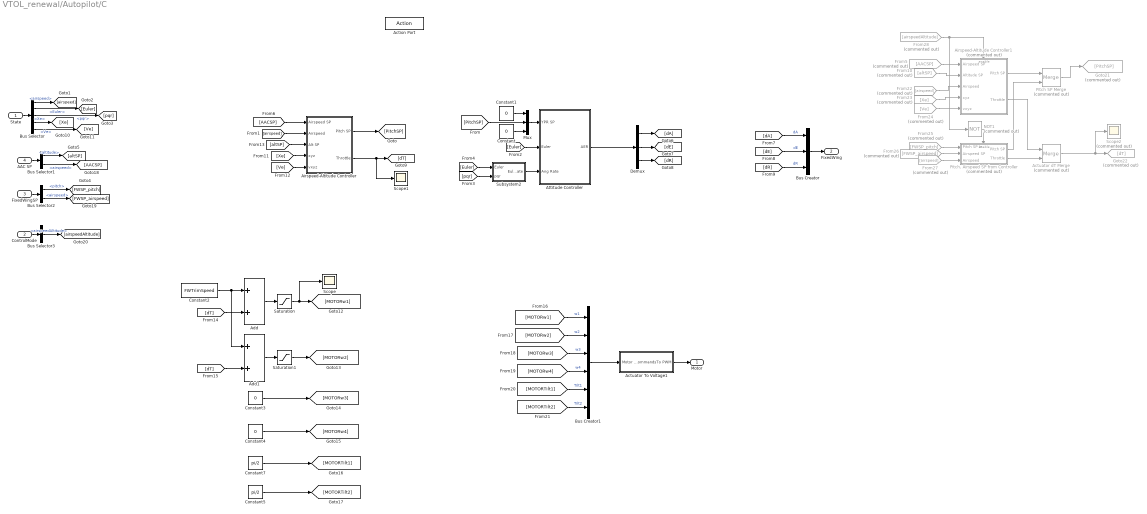
== system VTOL_renewal/Autopilot/C ==
  State : Inport
  ControlMode : Inport  Port=2
  FixedWingSP : Inport  Port=3
  AAC SP : Inport  Port=4
  Action Port : ActionPort  ActionPortLabel=case [ FixedWing ]:
  Actuator To Voltage1 : Subsystem
  Actuator dT Merge : Merge  Commented=on
  Add : Sum
  Add1 : Sum
  Airspeed-Altitude Controller : Subsystem
  Airspeed-Altitude Controller1 : Subsystem  Commented=on
  Attitude Controller : Subsystem
  Bus Creator : BusCreator  Inputs=3
  Bus Creator1 : BusCreator  Inputs=6
  Bus Selector : BusSelector  OutputSignals=airspeed,Euler,pqr,Xe,Ve
  Bus Selector1 : BusSelector  OutputSignals=altitude,airspeed
  Bus Selector2 : BusSelector  OutputSignals=pitch,airspeed
  Bus Selector3 : BusSelector  OutputSignals=airspeedAltitude
  Constant{,1,3..4} (4 alike) : Constant  Value=0
  Constant2 : Constant  Value=FWTrimSpeed
  Constant5 : Constant  Value=pi/2
  Constant7 : Constant  Value=pi/2
  Demux : Demux  Outputs=3
  From10 : From  Commented=on  GotoTag=altSP
  From22 : From  Commented=on  GotoTag=airspeed
  From23 : From  Commented=on  GotoTag=Xe
  From24 : From  Commented=on  GotoTag=Ve
  From25 : From  Commented=on  GotoTag=FWSP_pitch
  From26 : From  Commented=on  GotoTag=FWSP_airspeed
  From27 : From  Commented=on  GotoTag=airspeed
  From28 : From  Commented=on  GotoTag=airspeedAltitude
  From5 : From  Commented=on  GotoTag=AACSP
  Goto21 : Goto  Commented=on  GotoTag=PitchSP
  Goto22 : Goto  Commented=on  GotoTag=dT
  Mux : Mux  Inputs=3
  NOT1 : Logic  Commented=on  Operator=NOT  IconShape=distinctive  AllPortsSameDT=off  OutDataTypeStr=boolean
  Pitch SP Merge : Merge  Commented=on
  "Pitch, Airspeed SP from Controller" : Subsystem  Commented=on  TreatAsAtomicUnit=on
  Saturation : Saturate  UpperLimit=Inf  LowerLimit=0
  Saturation1 : Saturate  UpperLimit=Inf  LowerLimit=0
  Scope : Scope
  Scope1 : Scope
  Scope2 : Scope  Commented=on
  Subsystem2 : Subsystem
  Motor : Outport
  FixedWing : Outport  Port=2
  wires:
  [pqr] -> Subsystem2/2(pqr)
  Mux/1 -> Attitude Controller/1(YPR SP)
  Attitude Controller/1(AER) -> Demux/1
  Subsystem2/1(Euler Rate) -> Attitude Controller/3(Ang Rate)
  Demux/1 -> [dA]
  [AACSP] -> Airspeed-Altitude Controller/1(Airspeed SP)
  Demux/3 -> [dR]
  [airspeed] -> Airspeed-Altitude Controller/2(Airspeed)
  Constant1/1 -> Mux/1
  [Euler] -> Subsystem2/1(Euler)
  Demux/2 -> [dE]
  Constant/1 -> Mux/3
  [PitchSP] -> Mux/2
  State/1 -> Bus Selector/1
  Bus Selector/1 -> [airspeed]  "<airspeed>"
  Bus Selector/2 -> [Euler]  "<Euler>"
  Bus Selector/3 -> [pqr]  "<pqr>"
  [Euler] -> Attitude Controller/2(Euler)
  Bus Creator/1 -> FixedWing/1
  [dR] -> Bus Creator/3  "dR"
  [dE] -> Bus Creator/2  "dE"
  [dA] -> Bus Creator/1  "dA"
  Bus Selector/4 -> [Xe]  "<Xe>"
  Bus Selector/5 -> [Ve]  "<Ve>"
  [Xe] -> Airspeed-Altitude Controller/4(xyz)
  [Ve] -> Airspeed-Altitude Controller/5(vxyz)
  AAC SP/1 -> Bus Selector1/1
  Bus Selector1/1 -> [altSP]  "<altitude>"
  [altSP] -> Airspeed-Altitude Controller/3(Alt SP)
  Constant4/1 -> [MOTORw4]
  Saturation/1 -> [MOTORw1], Scope/1
  Add1/1 -> Saturation1/1
  Constant3/1 -> [MOTORw3]
  [dT] -> Add1/2
  Saturation1/1 -> [MOTORw2]
  Constant2/1 -> Add/1, Add1/1
  [dT] -> Add/2
  Add/1 -> Saturation/1
  Bus Creator1/1 -> Actuator To Voltage1/1(Motor Commands)
  [MOTORw1] -> Bus Creator1/1  "w1"
  [MOTORw2] -> Bus Creator1/2  "w2"
  [MOTORw3] -> Bus Creator1/3  "w3"
  [MOTORw4] -> Bus Creator1/4  "w4"
  [MOTORTilt1] -> Bus Creator1/5  "Tilt1"
  [MOTORTilt2] -> Bus Creator1/6  "Tilt2"
  Actuator To Voltage1/1(To PWM) -> Motor/1
  Bus Selector1/2 -> [AACSP]  "<airspeed>"
  Airspeed-Altitude Controller/1(Pitch SP) -> [PitchSP]
  Constant7/1 -> [MOTORTilt1]
  Constant5/1 -> [MOTORTilt2]
  FixedWingSP/1 -> Bus Selector2/1
  Bus Selector2/1 -> [FWSP_pitch]  "<pitch>"
  Bus Selector2/2 -> [FWSP_airspeed]  "<airspeed>"
  ControlMode/1 -> Bus Selector3/1
  Bus Selector3/1 -> [airspeedAltitude]  "<airspeedAltitude>"
  From25/1 -> "Pitch, Airspeed SP from Controller"/1(Pitch SP In)
  From27/1 -> "Pitch, Airspeed SP from Controller"/3(Airspeed)
  From23/1 -> Airspeed-Altitude Controller1/4(xyz)
  From10/1 -> Airspeed-Altitude Controller1/2(Altitude SP)
  "Pitch, Airspeed SP from Controller"/2(Throttle) -> Actuator dT Merge/2
  "Pitch, Airspeed SP from Controller"/1(Pitch SP) -> Pitch SP Merge/2
  Airspeed-Altitude Controller1/2(Throttle) -> Actuator dT Merge/1
  From26/1 -> "Pitch, Airspeed SP from Controller"/2(Airspeed SP)
  From24/1 -> Airspeed-Altitude Controller1/5(vxyz)
  Airspeed-Altitude Controller1/1(Pitch SP) -> Pitch SP Merge/1
  Pitch SP Merge/1 -> Goto21/1
  From5/1 -> Airspeed-Altitude Controller1/1(Airspeed SP)
  From22/1 -> Airspeed-Altitude Controller1/3(Airspeed)
  NOT1/1 -> "Pitch, Airspeed SP from Controller"/Enable
  From28/1 -> Airspeed-Altitude Controller1/Enable, NOT1/1
  Actuator dT Merge/1 -> Goto22/1, Scope2/1
  Airspeed-Altitude Controller/2(Throttle) -> Scope1/1, [dT]

== system VTOL_renewal/Autopilot/Fixed Wing Controller ==
  States : Inport
  Control Mode : Inport  Port=2
  AAC SP : Inport  Port=3
  FixedWingSP : Inport  Port=4
  AERT : Inport  Port=5
  Fixed Wing Controller Simulation : Subsystem  VariantControl=TuningMode == 0
  Actuator : Outport

== system VTOL_renewal/Autopilot/Manual Control ==
  Bus Creator : BusCreator  Inputs=4
  Constant{,1..3} (4 alike) : Constant  Value=0
  AERT : Outport
  wires:
  Constant/1 -> Bus Creator/1  "aileron"
  Constant1/1 -> Bus Creator/2  "throttle"
  Constant2/1 -> Bus Creator/3  "elevator"
  Constant3/1 -> Bus Creator/4  "rudder"
  Bus Creator/1 -> AERT/1

== system VTOL_renewal/Autopilot/Scheduler ==
  MotorCommands : Inport
  TiltSchedule : Inport  Port=2
  FlightState : Inport  Port=3  OutDataTypeStr=Enum: flightState
  States : Inport  Port=4
  TransitionDone : Inport  Port=5
  FixedWingActuators : Inport  Port=6
  Subsystem : Subsystem  ReferencedSubsystem=FixedWingScheduler
  Subsystem1 : Subsystem  ReferencedSubsystem=MulticopterScheduler
  MotorActuatorCommands : Outport
  CtrlSurfaceCommands : Outport  Port=2  VectorParamsAs1DForOutWhenUnconnected=off
  wires:
  Subsystem/1 -> Subsystem1/2, CtrlSurfaceCommands/1
  FlightState/1 -> Subsystem/1, Subsystem1/1  "Flight State"
  TiltSchedule/1 -> Subsystem1/4
  Subsystem1/1 -> MotorActuatorCommands/1
  MotorCommands/1 -> Subsystem1/3
  FixedWingActuators/1 -> Subsystem/2
  TransitionDone/1 -> Subsystem/3, Subsystem1/5  "Transition Done"
  States/1 -> Subsystem1/6

== system VTOL_renewal/Autopilot/Subsystem5 ==
  Ref : Inport
  States : Inport  Port=2
  Action Port : ActionPort
  Airspeed-Altitude : Subsystem
  Attitude : Subsystem
  Bus Creator : BusCreator  Inputs=6
  Constant{,3..7} (6 alike) : Constant  Value=0
  Constant1 : Constant  Value=25
  Constant2 : Constant
  Terminator : Terminator
  Motor : Outport
  FixedWing : Outport  Port=2
  wires:
  Ref/1 -> Airspeed-Altitude/1(Z Ref)
  States/1 -> Airspeed-Altitude/2(States), Attitude/1(States)
  Airspeed-Altitude/2(Throttle) -> Terminator/1
  Constant1/1 -> Airspeed-Altitude/3(Airspeed SP)
  Constant2/1 -> Airspeed-Altitude/4(Climb Rate SP)
  Airspeed-Altitude/1(Pitch SP) -> Attitude/2(Pitch SP)
  Attitude/1(AER) -> FixedWing/1
  Constant/1 -> Bus Creator/1  "w1"
  Constant3/1 -> Bus Creator/2  "w2"
  Constant4/1 -> Bus Creator/3  "w3"
  Constant5/1 -> Bus Creator/4  "w4"
  Constant6/1 -> Bus Creator/5  "Tilt1"
  Constant7/1 -> Bus Creator/6  "Tilt2"
  Bus Creator/1 -> Motor/1

== system VTOL_renewal/Autopilot/Tilt Scheduler ==
  note: Forward Transition Tilt Mode Manager
  note: Back Transition Tilt Mode Manager
  FlightMode : Inport
  States : Inport  Port=2
  Back Transition Scheduler : Subsystem
  Forward Transition Scheduler : Subsystem
  TiltAngle : Outport
  FlightState : Outport  Port=2
  wires:
  States/1 -> Back Transition Scheduler/3(States)
  Back Transition Scheduler/1(TiltAngle) -> TiltAngle/1
  FlightMode/1 -> Back Transition Scheduler/2(FlightMode), Forward Transition Scheduler/1(FlightMode)
  Forward Transition Scheduler/1(FlightState) -> FlightState/1
  Forward Transition Scheduler/2(Tilt Schedule) -> Back Transition Scheduler/1(Tilt Schedule)

== system VTOL_renewal/Digital Twin/Force and Moments ==
  Actuator : Inport
  CtrlSurfaces : Inport  Port=2
  States : Inport  Port=3
  Add : Sum  Inputs=++++
  Add1 : Sum
  AeroSwitch : Constant
  Aerodynamic Drag : Subsystem
  Aerodynamic Forces : Subsystem
  Bus Selector : BusSelector  OutputSignals=DCMbe,Vb
  Bus Selector3 : BusSelector  OutputSignals=Xe,Euler
  Constant4 : Constant  Value=0
  Constant5 : Constant  Value=0
  Gravity : Subsystem
  Propulsion : Subsystem
  Switch : Switch  Criteria=u2 > Threshold  SaturateOnIntegerOverflow=off  InputSameDT=off
  Switch1 : Switch  Criteria=u2 > Threshold  SaturateOnIntegerOverflow=off  InputSameDT=off
  Weather Model : Subsystem  Variant=on  VariantControl=Weather Model
  F : Outport
  M : Outport  Port=2
  RotorParams : Outport  Port=3
  AirData : Outport  Port=4
  wires:
  Bus Selector/1 -> Gravity/1(DCM_be), Aerodynamic Drag/1(DCM_be)  "<DCMbe>"
  Propulsion/3(F) -> Add/1
  Gravity/1(F_g) -> Add/2  "Gravity Force"
  Aerodynamic Drag/1(F_d) -> Add/4  "Drag Force"
  Bus Selector/2 -> Aerodynamic Drag/2(Vb)  "<Vb>"
  Add/1 -> F/1
  States/1 -> Bus Selector3/1, Bus Selector/1, Aerodynamic Forces/4(UAVState), Propulsion/2(States)  "States"
  CtrlSurfaces/1 -> Aerodynamic Forces/3(CtrlSurfaces)
  Add1/1 -> M/1
  Propulsion/2(M) -> Add1/2
  [AeroForce] -> Add/3  "Aerodynamic Force"
  Aerodynamic Forces/2(F) -> Switch/1
  Switch/1 -> [AeroForce]
  Constant4/1 -> Switch/3
  AeroSwitch/1 -> Switch/2, Switch1/2
  Constant5/1 -> Switch1/3
  Switch1/1 -> Add1/1, [AeroMoment]
  Aerodynamic Forces/3(M) -> Switch1/1
  Actuator/1 -> Propulsion/1(Actuator)
  Propulsion/1(RotorParameters) -> RotorParams/1
  Aerodynamic Forces/1(AirData) -> AirData/1, Weather Model/1(AirData)  "Air Data"
  Bus Selector3/1 -> Weather Model/2(Xe)  "<Xe>"
  Bus Selector3/2 -> Weather Model/3(Euler)  "<Euler>"
  Weather Model/1(Wind_e) -> Aerodynamic Forces/1(Wind_e)
  Weather Model/2(Rho) -> Aerodynamic Forces/2(Rho)
